simulink library "inp"  (R2021b)
settings: Solver=VariableStepAuto  StartTime=0.0  StopTime=10.0  RelTol=1e-3
undefined symbols (not defined in the file): C_TASK_5MS_S, FALSE, KINP_AcoreReadyToSlp_flg_ovrdflg, KINP_AcoreReadyToSlp_flg_ovrdval, KINP_AllowMovThd_OTA_enum_ovrdflg, KINP_AllowMovThd_OTA_enum_ovrdval, KINP_APSAngleTarget_Deg_ovrdflg, KINP_APSAngleTarget_Deg_ovrdval, KINP_APSDecReq_mps2_ovrdflg, KINP_APSDecReq_mps2_ovrdval, KINP_APSDecReqA_flg_ovrdflg, KINP_APSDecReqA_flg_ovrdval, KINP_APSDFLL_cm_ovrdflg, KINP_APSDFLL_cm_ovrdval, KINP_APSDFLR_cm_ovrdflg, KINP_APSDFLR_cm_ovrdval, KINP_APSDRLL_cm_ovrdflg, KINP_APSDRLL_cm_ovrdval, KINP_APSDRLR_cm_ovrdflg, KINP_APSDRLR_cm_ovrdval, KINP_APSExitCondition_enum_ovrdflg, KINP_APSExitCondition_enum_ovrdval, KINP_APSHWVer_enum_ovrdflg, KINP_APSHWVer_enum_ovrdval, KINP_APSProgressPCT_pct_ovrdflg, KINP_APSProgressPCT_pct_ovrdval, KINP_APSReq_enum_ovrdflg, KINP_APSReq_enum_ovrdval, KINP_APSRQDisplay_enum_ovrdflg, KINP_APSRQDisplay_enum_ovrdval, KINP_APSRqEPASCtrl_flg_ovrdflg, KINP_APSRqEPASCtrl_flg_ovrdval, KINP_APSShiftPosnReq_enum_ovrdval, KINP_APSShiftPosnReq_enum_ovrflg, KINP_APSSpeedCMD_kph_ovrdval, KINP_APSSpeedCMD_kph_ovrflg, KINP_APSStaSystem_enum_ovrdflg, KINP_APSStaSystem_enum_ovrdval, KINP_APSSWVer_enum_ovrdflg, KINP_APSSWVer_enum_ovrdval, KINP_APSVMCReqA_flg_ovrdval, KINP_APSVMCReqA_flg_ovrflg, KINP_APSVRqEPASCtrl_flg_ovrdflg, KINP_APSVRqEPASCtrl_flg_ovrdval, KINP_AuxBattVolmV_mV_ovrdflg, KINP_AuxBattVolmV_mV_ovrdval, KINP_CAASSta_enum_ovrdflg, KINP_CAASSta_enum_ovrdval, KINP_CAASVMCReqA_flg_ovrdval, KINP_CAASVMCReqA_flg_ovrflg, KINP_Chime_enum_ovrdflg, KINP_Chime_enum_ovrdval, KINP_ClearDTCcmd_flg_ovrdflg, KINP_ClearDTCcmd_flg_ovrdval, KINP_EvccAplusPwrUpReq_flg_ovrdflg, KINP_EvccAplusPwrUpReq_flg_ovrdval, KINP_LFID_raw_ovrdval, KINP_LFID_raw_ovrflg, KINP_LRID_raw_ovrdval, KINP_MemOffsetAccX_raw16_ovrdflg ... (+118)
libraries: FVT_lib x503, hcu_lib x1
(part 5 of 16)

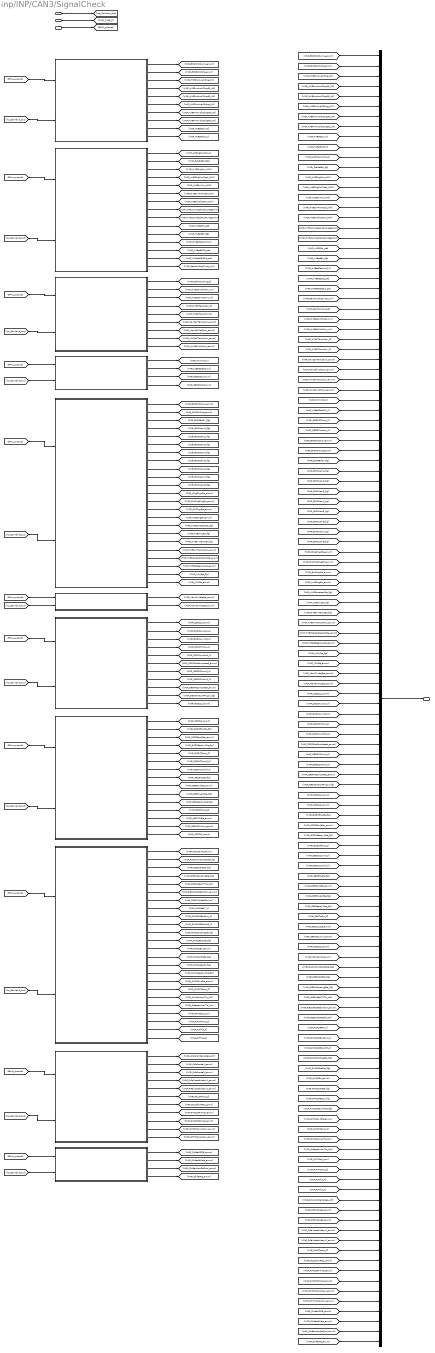
== system inp/INP/CAN3/SignalCheck ==
  inp_CanValid_bus : Inport
  TASK_TIME_S : Inport  Port=2
  BHAL_outputs : Inport  Port=3
  BMS1 : Subsystem
  BMS3 : Subsystem
  BMS4 : Subsystem
  BMS5 : Subsystem
  BMS6 : Subsystem
  BMS8 : Subsystem
  CCU1 : Subsystem
  CCU2 : Subsystem
  MCU_B_R1 : Subsystem
  MCU_B_R2 : Subsystem
  Shifter1 : Subsystem
  bus_creator : BusCreator  Inputs=128
  inp_Hal_bus : Outport
  wires:
  inp_CanValid_bus/1 -> [inp_CanValid_bus]
  TASK_TIME_S/1 -> [TASK_TIME_S]
  BHAL_outputs/1 -> [BHAL_outputs]
  [BHAL_outputs] -> BMS1/1(BHAL_outputs)
  [inp_CanValid_bus] -> BMS1/2(inp_CanValid_bus)
  BMS1/1(VINP_BMSChckSum1_enum) -> [VINP_BMSChckSum1_enum]
  BMS1/2(VINP_BMSRolCnct1_enum) -> [VINP_BMSRolCnct1_enum]
  BMS1/3(VINP_HVBPwrAvailChrg_kW) -> [VINP_HVBPwrAvailChrg_kW]
  BMS1/4(VINP_HVBPwrAvailChrg30_kW) -> [VINP_HVBPwrAvailChrg30_kW]
  BMS1/5(VINP_HVBPwrAvailChrg60_kW) -> [VINP_HVBPwrAvailChrg60_kW]
  BMS1/6(VINP_HVBPwrAvailDchrg_kW) -> [VINP_HVBPwrAvailDchrg_kW]
  BMS1/7(VINP_HVBPwrAvailDchrg30_kW) -> [VINP_HVBPwrAvailDchrg30_kW]
  BMS1/8(VINP_HVBPwrAvailDchrg60_kW) -> [VINP_HVBPwrAvailDchrg60_kW]
  BMS1/9(VINP_HVBattCurr_A) -> [VINP_HVBattCurr_A]
  BMS1/10(VINP_HVBattVolt_V) -> [VINP_HVBattVolt_V]
  [BHAL_outputs] -> BMS3/1(BHAL_outputs)
  [inp_CanValid_bus] -> BMS3/2(inp_CanValid_bus)
  BMS3/1(VINP_ACChrgCurrDis_A) -> [VINP_ACChrgCurrDis_A]
  BMS3/2(VINP_FireDetErr_flg) -> [VINP_FireDetErr_flg]
  BMS3/3(VINP_HVBChrgPwr_kWh) -> [VINP_HVBChrgPwr_kWh]
  BMS3/4(VINP_HVBChrgPwrTotal_kWh) -> [VINP_HVBChrgPwrTotal_kWh]
  BMS3/5(VINP_HVBDrvPwr_kWh) -> [VINP_HVBDrvPwr_kWh]
  BMS3/6(VINP_HVBDrvPwrTotal_kWh) -> [VINP_HVBDrvPwrTotal_kWh]
  BMS3/7(VINP_HVBFullChrgPwr_kWh) -> [VINP_HVBFullChrgPwr_kWh]
  BMS3/8(VINP_HVBIsoImpedenceN_Megaohm) -> [VINP_HVBIsoImpedenceN_Megaohm]
  BMS3/9(VINP_HVBIsoImpedenceP_Megaohm) -> [VINP_HVBIsoImpedenceP_Megaohm]
  BMS3/10(VINP_HVBSOH_pct) -> [VINP_HVBSOH_pct]
  BMS3/11(VINP_HVBattErr_flg) -> [VINP_HVBattErr_flg]
  BMS3/12(VINP_HVBattPackVolt_V) -> [VINP_HVBattPackVolt_V]
  BMS3/13(VINP_HVBattSOC_pct) -> [VINP_HVBattSOC_pct]
  BMS3/14(VINP_HVBattSOCDis_pct) -> [VINP_HVBattSOCDis_pct]
  BMS3/15(VINP_RemainChrgTime_min) -> [VINP_RemainChrgTime_min]
  [BHAL_outputs] -> BMS4/1(BHAL_outputs)
  [inp_CanValid_bus] -> BMS4/2(inp_CanValid_bus)
  BMS4/1(VINP_CellTempAvg_C) -> [VINP_CellTempAvg_C]
  BMS4/2(VINP_HVBCellVoltMax_mV) -> [VINP_HVBCellVoltMax_mV]
  BMS4/3(VINP_HVBCellVoltMin_mV) -> [VINP_HVBCellVoltMin_mV]
  BMS4/4(VINP_HVBMTempMax_C) -> [VINP_HVBMTempMax_C]
  BMS4/5(VINP_HVBMTempMin_C) -> [VINP_HVBMTempMin_C]
  BMS4/6(VINP_MaxCellTempNum_enum) -> [VINP_MaxCellTempNum_enum]
  BMS4/7(VINP_MaxCellVoltNum_enum) -> [VINP_MaxCellVoltNum_enum]
  BMS4/8(VINP_MinCellTempNum_enum) -> [VINP_MinCellTempNum_enum]
  BMS4/9(VINP_MinCellVoltNum_enum) -> [VINP_MinCellVoltNum_enum]
  [BHAL_outputs] -> BMS5/1(BHAL_outputs)
  [inp_CanValid_bus] -> BMS5/2(inp_CanValid_bus)
  BMS5/1(VINP_HVInVolt_V) -> [VINP_HVInVolt_V]
  BMS5/2(VINP_LVBattDet12V_V) -> [VINP_LVBattDet12V_V]
  BMS5/3(VINP_OBCDCCurLm_A) -> [VINP_OBCDCCurLm_A]
  BMS5/4(VINP_OBCDCVoltLm_V) -> [VINP_OBCDCVoltLm_V]
  [BHAL_outputs] -> BMS6/1(BHAL_outputs)
  [inp_CanValid_bus] -> BMS6/2(inp_CanValid_bus)
  BMS6/1(VINP_BMSChckSum_enum) -> [VINP_BMSChckSum_enum]
  BMS6/2(VINP_BMSRolCnct_enum) -> [VINP_BMSRolCnct_enum]
  BMS6/3(VINP_BMSREADY_flg) -> [VINP_BMSREADY_flg]
  BMS6/4(VINP_BMSWarn1_flg) -> [VINP_BMSWarn1_flg]
  BMS6/5(VINP_BMSWarn2_flg) -> [VINP_BMSWarn2_flg]
  BMS6/6(VINP_BMSWarn3_flg) -> [VINP_BMSWarn3_flg]
  BMS6/7(VINP_BMSWarn4_flg) -> [VINP_BMSWarn4_flg]
  BMS6/8(VINP_BMSWarn5_flg) -> [VINP_BMSWarn5_flg]
  BMS6/9(VINP_BMSWarn6_flg) -> [VINP_BMSWarn6_flg]
  BMS6/10(VINP_BMSWarn7_flg) -> [VINP_BMSWarn7_flg]
  BMS6/11(VINP_BMSWarn8_flg) -> [VINP_BMSWarn8_flg]
  BMS6/12(VINP_ChrgPlugSta_enum) -> [VINP_ChrgPlugSta_enum]
  BMS6/13(VINP_DisChrgPlugErr_enum) -> [VINP_DisChrgPlugErr_enum]
  BMS6/14(VINP_ExtChrgSta_enum) -> [VINP_ExtChrgSta_enum]
  BMS6/15(VINP_HVBChrgErr_enum) -> [VINP_HVBChrgErr_enum]
  BMS6/16(VINP_HVBContactorSta_flg) -> [VINP_HVBContactorSta_flg]
  BMS6/17(VINP_HVBHVILErr_flg) -> [VINP_HVBHVILErr_flg]
  BMS6/18(VINP_HVBOvrTempErr_flg) -> [VINP_HVBOvrTempErr_flg]
  BMS6/19(VINP_HVBOvrTempWarn_enum) -> [VINP_HVBOvrTempWarn_enum]
  BMS6/20(VINP_HVBPreheatPrecoolSta_enum) -> [VINP_HVBPreheatPrecoolSta_enum]
  BMS6/21(VINP_HVBattReady4Pre_enum) -> [VINP_HVBattReady4Pre_enum]
  BMS6/22(VINP_HVILSta_flg) -> [VINP_HVILSta_flg]
  BMS6/23(VINP_V2LSta_enum) -> [VINP_V2LSta_enum]
  [BHAL_outputs] -> BMS8/1(BHAL_outputs)
  [inp_CanValid_bus] -> BMS8/2(inp_CanValid_bus)
  BMS8/1(VINP_MainRlyNegSta_enum) -> [VINP_MainRlyNegSta_enum]
  BMS8/2(VINP_MainRlyPosSta_enum) -> [VINP_MainRlyPosSta_enum]
  [BHAL_outputs] -> CCU1/1(BHAL_outputs)
  [inp_CanValid_bus] -> CCU1/2(inp_CanValid_bus)
  CCU1/1(VINP_CSCCU1_enum) -> [VINP_CSCCU1_enum]
  CCU1/2(VINP_DCDCAuxCur_A) -> [VINP_DCDCAuxCur_A]
  CCU1/3(VINP_DCDCAuxVolt_V) -> [VINP_DCDCAuxVolt_V]
  CCU1/4(VINP_DCDCHVCur_A) -> [VINP_DCDCHVCur_A]
  CCU1/5(VINP_DCDCInVoltInf_V) -> [VINP_DCDCInVoltInf_V]
  CCU1/6(VINP_DCDCPreCompleted_enum) -> [VINP_DCDCPreCompleted_enum]
  CCU1/7(VINP_OBCDCCurrInf_A) -> [VINP_OBCDCCurrInf_A]
  CCU1/8(VINP_OBCDCVoltInf_V) -> [VINP_OBCDCVoltInf_V]
  CCU1/9(VINP_OBCPreCompleted_enum) -> [VINP_OBCPreCompleted_enum]
  CCU1/10(VINP_OBCWakeup4Plugin_flg) -> [VINP_OBCWakeup4Plugin_flg]
  CCU1/11(VINP_RCCCU1_enum) -> [VINP_RCCCU1_enum]
  [BHAL_outputs] -> CCU2/1(BHAL_outputs)
  [inp_CanValid_bus] -> CCU2/2(inp_CanValid_bus)
  CCU2/1(VINP_CSCCU2_enum) -> [VINP_CSCCU2_enum]
  CCU2/2(VINP_DCDCEnaSta_flg) -> [VINP_DCDCEnaSta_flg]
  CCU2/3(VINP_DCDCFaultSta_enum) -> [VINP_DCDCFaultSta_enum]
  CCU2/4(VINP_DCDCReady4Pre_flg) -> [VINP_DCDCReady4Pre_flg]
  CCU2/5(VINP_DCDCTemp_C) -> [VINP_DCDCTemp_C]
  CCU2/6(VINP_OBCACCurrInf_A) -> [VINP_OBCACCurrInf_A]
  CCU2/7(VINP_OBCACVoltInf_V) -> [VINP_OBCACVoltInf_V]
  CCU2/8(VINP_OBCEnaSta_flg) -> [VINP_OBCEnaSta_flg]
  CCU2/9(VINP_OBCFaultSta_enum) -> [VINP_OBCFaultSta_enum]
  CCU2/10(VINP_OBCPluginSta_flg) -> [VINP_OBCPluginSta_flg]
  CCU2/11(VINP_OBCReady4Pre_flg) -> [VINP_OBCReady4Pre_flg]
  CCU2/12(VINP_OBCTemp_C) -> [VINP_OBCTemp_C]
  CCU2/13(VINP_OBCV2LSta_enum) -> [VINP_OBCV2LSta_enum]
  CCU2/14(VINP_OBCACCurLim_enum) -> [VINP_OBCACCurLim_enum]
  CCU2/15(VINP_RCCCU2_enum) -> [VINP_RCCCU2_enum]
  [BHAL_outputs] -> MCU_B_R1/1(BHAL_outputs)
  [inp_CanValid_bus] -> MCU_B_R1/2(inp_CanValid_bus)
  MCU_B_R1/1(VINP_MCUWarnR_enum) -> [VINP_MCUWarnR_enum]
  MCU_B_R1/2(VINP_RrActvDmpDisabSta_flg) -> [VINP_RrActvDmpDisabSta_flg]
  MCU_B_R1/3(VINP_RrEDUDrtSta_flg) -> [VINP_RrEDUDrtSta_flg]
  MCU_B_R1/4(VINP_RrEDUOpratingSta_flg) -> [VINP_RrEDUOpratingSta_flg]
  MCU_B_R1/5(VINP_RrEDURealTMTq_Nm) -> [VINP_RrEDURealTMTq_Nm]
  MCU_B_R1/6(VINP_RrEDURotateDirction_enum) -> [VINP_RrEDURotateDirction_enum]
  MCU_B_R1/7(VINP_RrEDUTqReqFbk_Nm) -> [VINP_RrEDUTqReqFbk_Nm]
  MCU_B_R1/8(VINP_RrMCUBAT_V) -> [VINP_RrMCUBAT_V]
  MCU_B_R1/9(VINP_RrMCUDCBusCurr_A) -> [VINP_RrMCUDCBusCurr_A]
  MCU_B_R1/10(VINP_RrMCUDCBusVolt_V) -> [VINP_RrMCUDCBusVolt_V]
  MCU_B_R1/11(VINP_RrMCUDischrgSta_flg) -> [VINP_RrMCUDischrgSta_flg]
  MCU_B_R1/12(VINP_RrMCUEnaSta_flg) -> [VINP_RrMCUEnaSta_flg]
  MCU_B_R1/13(VINP_RrMCUErr_enum) -> [VINP_RrMCUErr_enum]
  MCU_B_R1/14(VINP_RrMCUIGNsta_flg) -> [VINP_RrMCUIGNsta_flg]
  MCU_B_R1/15(VINP_RrMCUReady_flg) -> [VINP_RrMCUReady_flg]
  MCU_B_R1/16(VINP_RrMCUReady4Pre_flg) -> [VINP_RrMCUReady4Pre_flg]
  MCU_B_R1/17(VINP_RrMCUSysSta_enum) -> [VINP_RrMCUSysSta_enum]
  MCU_B_R1/18(VINP_RrMCUTemp_C) -> [VINP_RrMCUTemp_C]
  MCU_B_R1/19(VINP_RrMotorAvailTq_Nm) -> [VINP_RrMotorAvailTq_Nm]
  MCU_B_R1/20(VINP_RrRegenAvailTq_Nm) -> [VINP_RrRegenAvailTq_Nm]
  MCU_B_R1/21(VINP_RrTMSpd_rpm) -> [VINP_RrTMSpd_rpm]
  MCU_B_R1/22(VINP_RrTMTemp_C) -> [VINP_RrTMTemp_C]
  MCU_B_R1/23(VINP_RrTMid_A) -> [VINP_RrTMid_A]
  MCU_B_R1/24(VINP_RrTMiq_A) -> [VINP_RrTMiq_A]
  [BHAL_outputs] -> MCU_B_R2/1(BHAL_outputs)
  [inp_CanValid_bus] -> MCU_B_R2/2(inp_CanValid_bus)
  MCU_B_R2/1(VINP_RrCoolanttempReq_cnt) -> [VINP_RrCoolanttempReq_cnt]
  MCU_B_R2/2(VINP_RrFailcode1_enum) -> [VINP_RrFailcode1_enum]
  MCU_B_R2/3(VINP_RrFailcode2_enum) -> [VINP_RrFailcode2_enum]
  MCU_B_R2/4(VINP_RrFailcodehistory1_enum) -> [VINP_RrFailcodehistory1_enum]
  MCU_B_R2/5(VINP_RrFailcodehistory2_enum) -> [VINP_RrFailcodehistory2_enum]
  MCU_B_R2/6(VINP_RrLLCTemp_C) -> [VINP_RrLLCTemp_C]
  MCU_B_R2/7(VINP_RrLLCflowReq_Lpmin) -> [VINP_RrLLCflowReq_Lpmin]
  MCU_B_R2/8(VINP_RrMCU3HWVer_enum) -> [VINP_RrMCU3HWVer_enum]
  MCU_B_R2/9(VINP_RrMCU3SWVer_enum) -> [VINP_RrMCU3SWVer_enum]
  MCU_B_R2/10(VINP_RrMCUTempWarn_enum) -> [VINP_RrMCUTempWarn_enum]
  MCU_B_R2/11(VINP_RrTMTempWarn_enum) -> [VINP_RrTMTempWarn_enum]
  [BHAL_outputs] -> Shifter1/1(BHAL_outputs)
  [inp_CanValid_bus] -> Shifter1/2(inp_CanValid_bus)
  Shifter1/1(VINP_ShifterCRC8_enum) -> [VINP_ShifterCRC8_enum]
  Shifter1/2(VINP_ShifterFailsta_enum) -> [VINP_ShifterFailsta_enum]
  Shifter1/3(VINP_ShifterHandleCmd_enum) -> [VINP_ShifterHandleCmd_enum]
  Shifter1/4(VINP_ShifterRC_enum) -> [VINP_ShifterRC_enum]
  bus_creator/1 -> inp_Hal_bus/1
  [VINP_BMSChckSum1_enum] -> bus_creator/1
  [VINP_BMSRolCnct1_enum] -> bus_creator/2
  [VINP_HVBPwrAvailChrg_kW] -> bus_creator/3
  [VINP_HVBPwrAvailChrg30_kW] -> bus_creator/4
  [VINP_HVBPwrAvailChrg60_kW] -> bus_creator/5
  [VINP_HVBPwrAvailDchrg_kW] -> bus_creator/6
  [VINP_HVBPwrAvailDchrg30_kW] -> bus_creator/7
  [VINP_HVBPwrAvailDchrg60_kW] -> bus_creator/8
  [VINP_HVBattCurr_A] -> bus_creator/9
  [VINP_HVBattVolt_V] -> bus_creator/10
  [VINP_ACChrgCurrDis_A] -> bus_creator/11
  [VINP_FireDetErr_flg] -> bus_creator/12
  [VINP_HVBChrgPwr_kWh] -> bus_creator/13
  [VINP_HVBChrgPwrTotal_kWh] -> bus_creator/14
  [VINP_HVBDrvPwr_kWh] -> bus_creator/15
  [VINP_HVBDrvPwrTotal_kWh] -> bus_creator/16
  [VINP_HVBFullChrgPwr_kWh] -> bus_creator/17
  [VINP_HVBIsoImpedenceN_Megaohm] -> bus_creator/18
  [VINP_HVBIsoImpedenceP_Megaohm] -> bus_creator/19
  [VINP_HVBSOH_pct] -> bus_creator/20
  [VINP_HVBattErr_flg] -> bus_creator/21
  [VINP_HVBattPackVolt_V] -> bus_creator/22
  [VINP_HVBattSOC_pct] -> bus_creator/23
  [VINP_HVBattSOCDis_pct] -> bus_creator/24
  [VINP_RemainChrgTime_min] -> bus_creator/25
  [VINP_CellTempAvg_C] -> bus_creator/26
  [VINP_HVBCellVoltMax_mV] -> bus_creator/27
  [VINP_HVBCellVoltMin_mV] -> bus_creator/28
  [VINP_HVBMTempMax_C] -> bus_creator/29
  [VINP_HVBMTempMin_C] -> bus_creator/30
  [VINP_MaxCellTempNum_enum] -> bus_creator/31
  [VINP_MaxCellVoltNum_enum] -> bus_creator/32
  [VINP_MinCellTempNum_enum] -> bus_creator/33
  [VINP_MinCellVoltNum_enum] -> bus_creator/34
  [VINP_HVInVolt_V] -> bus_creator/35
  [VINP_LVBattDet12V_V] -> bus_creator/36
  [VINP_OBCDCCurLm_A] -> bus_creator/37
  [VINP_OBCDCVoltLm_V] -> bus_creator/38
  [VINP_BMSChckSum_enum] -> bus_creator/39
  [VINP_BMSRolCnct_enum] -> bus_creator/40
  [VINP_BMSREADY_flg] -> bus_creator/41
  [VINP_BMSWarn1_flg] -> bus_creator/42
  [VINP_BMSWarn2_flg] -> bus_creator/43
  [VINP_BMSWarn3_flg] -> bus_creator/44
  [VINP_BMSWarn4_flg] -> bus_creator/45
  [VINP_BMSWarn5_flg] -> bus_creator/46
  [VINP_BMSWarn6_flg] -> bus_creator/47
  [VINP_BMSWarn7_flg] -> bus_creator/48
  [VINP_BMSWarn8_flg] -> bus_creator/49
  [VINP_ChrgPlugSta_enum] -> bus_creator/50
  [VINP_DisChrgPlugErr_enum] -> bus_creator/51
  [VINP_ExtChrgSta_enum] -> bus_creator/52
  [VINP_HVBChrgErr_enum] -> bus_creator/53
  [VINP_HVBContactorSta_flg] -> bus_creator/54
  [VINP_HVBHVILErr_flg] -> bus_creator/55
  [VINP_HVBOvrTempErr_flg] -> bus_creator/56
  [VINP_HVBOvrTempWarn_enum] -> bus_creator/57
  [VINP_HVBPreheatPrecoolSta_enum] -> bus_creator/58
  [VINP_HVBattReady4Pre_enum] -> bus_creator/59
  [VINP_HVILSta_flg] -> bus_creator/60
  [VINP_V2LSta_enum] -> bus_creator/61
  [VINP_MainRlyNegSta_enum] -> bus_creator/62
  [VINP_MainRlyPosSta_enum] -> bus_creator/63
  [VINP_CSCCU1_enum] -> bus_creator/64
  [VINP_DCDCAuxCur_A] -> bus_creator/65
  [VINP_DCDCAuxVolt_V] -> bus_creator/66
  [VINP_DCDCHVCur_A] -> bus_creator/67
  [VINP_DCDCInVoltInf_V] -> bus_creator/68
  [VINP_DCDCPreCompleted_enum] -> bus_creator/69
  [VINP_OBCDCCurrInf_A] -> bus_creator/70
  [VINP_OBCDCVoltInf_V] -> bus_creator/71
  [VINP_OBCPreCompleted_enum] -> bus_creator/72
  [VINP_OBCWakeup4Plugin_flg] -> bus_creator/73
  [VINP_RCCCU1_enum] -> bus_creator/74
  [VINP_CSCCU2_enum] -> bus_creator/75
  [VINP_DCDCEnaSta_flg] -> bus_creator/76
  [VINP_DCDCFaultSta_enum] -> bus_creator/77
  [VINP_DCDCReady4Pre_flg] -> bus_creator/78
  [VINP_DCDCTemp_C] -> bus_creator/79
  [VINP_OBCACCurrInf_A] -> bus_creator/80
  [VINP_OBCACVoltInf_V] -> bus_creator/81
  [VINP_OBCEnaSta_flg] -> bus_creator/82
  [VINP_OBCFaultSta_enum] -> bus_creator/83
  [VINP_OBCPluginSta_flg] -> bus_creator/84
  [VINP_OBCReady4Pre_flg] -> bus_creator/85
  [VINP_OBCTemp_C] -> bus_creator/86
  [VINP_OBCV2LSta_enum] -> bus_creator/87
  [VINP_OBCACCurLim_enum] -> bus_creator/88
  [VINP_RCCCU2_enum] -> bus_creator/89
  [VINP_MCUWarnR_enum] -> bus_creator/90
  [VINP_RrActvDmpDisabSta_flg] -> bus_creator/91
  [VINP_RrEDUDrtSta_flg] -> bus_creator/92
  [VINP_RrEDUOpratingSta_flg] -> bus_creator/93
  [VINP_RrEDURealTMTq_Nm] -> bus_creator/94
  [VINP_RrEDURotateDirction_enum] -> bus_creator/95
  [VINP_RrEDUTqReqFbk_Nm] -> bus_creator/96
  [VINP_RrMCUBAT_V] -> bus_creator/97
  [VINP_RrMCUDCBusCurr_A] -> bus_creator/98
  [VINP_RrMCUDCBusVolt_V] -> bus_creator/99
  [VINP_RrMCUDischrgSta_flg] -> bus_creator/100
  [VINP_RrMCUEnaSta_flg] -> bus_creator/101
  [VINP_RrMCUErr_enum] -> bus_creator/102
  [VINP_RrMCUIGNsta_flg] -> bus_creator/103
  [VINP_RrMCUReady_flg] -> bus_creator/104
  [VINP_RrMCUReady4Pre_flg] -> bus_creator/105
  [VINP_RrMCUSysSta_enum] -> bus_creator/106
  [VINP_RrMCUTemp_C] -> bus_creator/107
  [VINP_RrMotorAvailTq_Nm] -> bus_creator/108
  [VINP_RrRegenAvailTq_Nm] -> bus_creator/109
  [VINP_RrTMSpd_rpm] -> bus_creator/110
  [VINP_RrTMTemp_C] -> bus_creator/111
  [VINP_RrTMid_A] -> bus_creator/112
  [VINP_RrTMiq_A] -> bus_creator/113
  [VINP_RrCoolanttempReq_cnt] -> bus_creator/114
  [VINP_RrFailcode1_enum] -> bus_creator/115
  [VINP_RrFailcode2_enum] -> bus_creator/116
  [VINP_RrFailcodehistory1_enum] -> bus_creator/117
  [VINP_RrFailcodehistory2_enum] -> bus_creator/118
  [VINP_RrLLCTemp_C] -> bus_creator/119
  [VINP_RrLLCflowReq_Lpmin] -> bus_creator/120
  [VINP_RrMCU3HWVer_enum] -> bus_creator/121
  [VINP_RrMCU3SWVer_enum] -> bus_creator/122
  [VINP_RrMCUTempWarn_enum] -> bus_creator/123
  [VINP_RrTMTempWarn_enum] -> bus_creator/124
  [VINP_ShifterCRC8_enum] -> bus_creator/125
  [VINP_ShifterFailsta_enum] -> bus_creator/126
  [VINP_ShifterHandleCmd_enum] -> bus_creator/127
  [VINP_ShifterRC_enum] -> bus_creator/128

== system inp/INP/CAN4/CommunicationCheck ==
  BHAL_outputs : Inport
  CANMsgInvalidDKC1 : FVT_lib/inp/CAN_Msg_Validity_Process_template  SystemSampleTime=-1  VariantActivationTime=update diagram  Latency=0  AutoFrameSizeCalculation=off
      link override ovrdflg: Value=KINP_CANMsgInvalidDKC1_flg_ovrdflg
      link override ovrdval: Value=KINP_CANMsgInvalidDKC1_flg_ovrdval
  CANMsgInvalidDKC2 : FVT_lib/inp/CAN_Msg_Validity_Process_template  SystemSampleTime=-1  VariantActivationTime=update diagram  Latency=0  AutoFrameSizeCalculation=off
      link override ovrdflg: Value=KINP_CANMsgInvalidDKC2_flg_ovrdflg
      link override ovrdval: Value=KINP_CANMsgInvalidDKC2_flg_ovrdval
  CANMsgInvalidZ24C10000 : FVT_lib/inp/CAN_Msg_Validity_Process_template  SystemSampleTime=-1  VariantActivationTime=update diagram  Latency=0  AutoFrameSizeCalculation=off
      link override ovrdflg: Value=KINP_CANMsgInvalidZ24C10000_flg_ovrdflg
      link override ovrdval: Value=KINP_CANMsgInvalidZ24C10000_flg_ovrdval
  CANMsgInvalidZ24CE1000 : FVT_lib/inp/CAN_Msg_Validity_Process_template  SystemSampleTime=-1  VariantActivationTime=update diagram  Latency=0  AutoFrameSizeCalculation=off
      link override ovrdflg: Value=KINP_CANMsgInvalidZ24CE1000_flg_ovrdflg
      link override ovrdval: Value=KINP_CANMsgInvalidZ24CE1000_flg_ovrdval
  CANMsgInvalidZONEDR1 : FVT_lib/inp/CAN_Msg_Validity_Process_template  SystemSampleTime=-1  VariantActivationTime=update diagram  Latency=0  AutoFrameSizeCalculation=off
      link override ovrdflg: Value=KINP_CANMsgInvalidZONEDR1_flg_ovrdflg
      link override ovrdval: Value=KINP_CANMsgInvalidZONEDR1_flg_ovrdval
  CANMsgInvalidZONEDRVCU : FVT_lib/inp/CAN_Msg_Validity_Process_template  SystemSampleTime=-1  VariantActivationTime=update diagram  Latency=0  AutoFrameSizeCalculation=off
      link override ovrdflg: Value=KINP_CANMsgInvalidZONEDRVCU_flg_ovrdflg
      link override ovrdval: Value=KINP_CANMsgInvalidZONEDRVCU_flg_ovrdval
  CANMsgInvalidZONEFR1 : FVT_lib/inp/CAN_Msg_Validity_Process_template  SystemSampleTime=-1  VariantActivationTime=update diagram  Latency=0  AutoFrameSizeCalculation=off
      link override ovrdflg: Value=KINP_CANMsgInvalidZONEFR1_flg_ovrdflg
      link override ovrdval: Value=KINP_CANMsgInvalidZONEFR1_flg_ovrdval
  CANMsgInvalidZONEFRVCU : FVT_lib/inp/CAN_Msg_Validity_Process_template  SystemSampleTime=-1  VariantActivationTime=update diagram  Latency=0  AutoFrameSizeCalculation=off
      link override ovrdflg: Value=KINP_CANMsgInvalidZONEFRVCU_flg_ovrdflg
      link override ovrdval: Value=KINP_CANMsgInvalidZONEFRVCU_flg_ovrdval
  CANMsgInvalidzGWAPTC1 : FVT_lib/inp/CAN_Msg_Validity_Process_template  SystemSampleTime=-1  VariantActivationTime=update diagram  Latency=0  AutoFrameSizeCalculation=off
      link override ovrdflg: Value=KINP_CANMsgInvalidzGWAPTC1_flg_ovrdflg
      link override ovrdval: Value=KINP_CANMsgInvalidzGWAPTC1_flg_ovrdval
  CANMsgInvalidzGWCANFr1 : FVT_lib/inp/CAN_Msg_Validity_Process_template  SystemSampleTime=-1  VariantActivationTime=update diagram  Latency=0  AutoFrameSizeCalculation=off
      link override ovrdflg: Value=KINP_CANMsgInvalidzGWCANFr1_flg_ovrdflg
      link override ovrdval: Value=KINP_CANMsgInvalidzGWCANFr1_flg_ovrdval
  CANMsgInvalidzGWLINDr1 : FVT_lib/inp/CAN_Msg_Validity_Process_template  SystemSampleTime=-1  VariantActivationTime=update diagram  Latency=0  AutoFrameSizeCalculation=off
      link override ovrdflg: Value=KINP_CANMsgInvalidzGWLINDr1_flg_ovrdflg
      link override ovrdval: Value=KINP_CANMsgInvalidzGWLINDr1_flg_ovrdval
  bus_creator : BusCreator  Inputs=11
  bus_selector : BusSelector  OutputSignals=VHAL_CANMsgInvalidDKC1_flg,VHAL_CANMsgInvalidDKC2_flg,VHAL_CANMsgInvalidZ24C10000_flg,VHAL_CANMsgInvalidZ24CE1000_flg,VHAL_CANMsgInvalidZONEDR1_flg,VHAL_CANMsgInvalidZONEDRVCU_flg,VHAL_CANMsgInvalidZONEFR1_flg,VHAL_CANMsgInvalidZONEFRVCU_flg,VHAL_CANMsgInvalidzGWAPTC1_flg,VHAL_CANMsgInvalidzGWCANFr1_flg,VHAL_CANMsgInvalidzGWLINDr1_flg
  not{1..11} (11 alike) : Logic  Operator=NOT  AllPortsSameDT=off  OutDataTypeStr=boolean
  inp_CanValid_bus : Outport
  wires:
  BHAL_outputs/1 -> [BHAL_outputs]
  bus_selector/1 -> CANMsgInvalidDKC1/1  "<VHAL_CANMsgInvalidDKC1_flg>"
  CANMsgInvalidDKC1/1 -> not1/1
  not1/1 -> bus_creator/1  "VINP_CANMsgValidDKC1_flg"
  bus_selector/2 -> CANMsgInvalidDKC2/1  "<VHAL_CANMsgInvalidDKC2_flg>"
  CANMsgInvalidDKC2/1 -> not2/1
  not2/1 -> bus_creator/2  "VINP_CANMsgValidDKC2_flg"
  bus_selector/3 -> CANMsgInvalidZ24C10000/1  "<VHAL_CANMsgInvalidZ24C10000_flg>"
  CANMsgInvalidZ24C10000/1 -> not3/1
  not3/1 -> bus_creator/3  "VINP_CANMsgValidZ24C10000_flg"
  bus_selector/4 -> CANMsgInvalidZ24CE1000/1  "<VHAL_CANMsgInvalidZ24CE1000_flg>"
  CANMsgInvalidZ24CE1000/1 -> not4/1
  not4/1 -> bus_creator/4  "VINP_CANMsgValidZ24CE1000_flg"
  bus_selector/5 -> CANMsgInvalidZONEDR1/1  "<VHAL_CANMsgInvalidZONEDR1_flg>"
  CANMsgInvalidZONEDR1/1 -> not5/1
  not5/1 -> bus_creator/5  "VINP_CANMsgValidZONEDR1_flg"
  bus_selector/6 -> CANMsgInvalidZONEDRVCU/1  "<VHAL_CANMsgInvalidZONEDRVCU_flg>"
  CANMsgInvalidZONEDRVCU/1 -> not6/1
  not6/1 -> bus_creator/6  "VINP_CANMsgValidZONEDRVCU_flg"
  bus_selector/7 -> CANMsgInvalidZONEFR1/1  "<VHAL_CANMsgInvalidZONEFR1_flg>"
  CANMsgInvalidZONEFR1/1 -> not7/1
  not7/1 -> bus_creator/7  "VINP_CANMsgValidZONEFR1_flg"
  bus_selector/8 -> CANMsgInvalidZONEFRVCU/1  "<VHAL_CANMsgInvalidZONEFRVCU_flg>"
  CANMsgInvalidZONEFRVCU/1 -> not8/1
  not8/1 -> bus_creator/8  "VINP_CANMsgValidZONEFRVCU_flg"
  bus_selector/9 -> CANMsgInvalidzGWAPTC1/1  "<VHAL_CANMsgInvalidzGWAPTC1_flg>"
  CANMsgInvalidzGWAPTC1/1 -> not9/1
  not9/1 -> bus_creator/9  "VINP_CANMsgValidzGWAPTC1_flg"
  bus_selector/10 -> CANMsgInvalidzGWCANFr1/1  "<VHAL_CANMsgInvalidzGWCANFr1_flg>"
  CANMsgInvalidzGWCANFr1/1 -> not10/1
  not10/1 -> bus_creator/10  "VINP_CANMsgValidzGWCANFr1_flg"
  bus_selector/11 -> CANMsgInvalidzGWLINDr1/1  "<VHAL_CANMsgInvalidzGWLINDr1_flg>"
  CANMsgInvalidzGWLINDr1/1 -> not11/1
  not11/1 -> bus_creator/11  "VINP_CANMsgValidzGWLINDr1_flg"
  [BHAL_outputs] -> bus_selector/1
  bus_creator/1 -> inp_CanValid_bus/1

== system inp/INP/CAN4/CreateBus ==
  inp_CanValid_bus : Inport
  inp_Hal_bus : Inport  Port=2
  UnitConverter_{1..11,20,22,29..32,35..36,38..41,63..64,67..69,80,110,113,117..119,121..122,124..125,127..128,130..131,133..147} (57 alike) : DataTypeConversion  OutDataTypeStr=boolean
  UnitConverter_{12..19,21,37,43,45,47,49,51,53,55,57,59,61..62,70,72,74..79,82,84,86,88,90,92,94,96..100,102,111..112,114..116,132} (48 alike) : DataTypeConversion  OutDataTypeStr=uint8
  UnitConverter_{26..28,33..34,42,44,46,48,50,52,54,56,58,60,65..66,71,73,81,83,85,87,89,91,93,95,101,103..108,120,123,126,129} (38 alike) : DataTypeConversion  OutDataTypeStr=single
  UnitConverter_109 : DataTypeConversion  OutDataTypeStr=uint16
  UnitConverter_23 : DataTypeConversion  OutDataTypeStr=uint64
  UnitConverter_24 : DataTypeConversion  OutDataTypeStr=uint64
  UnitConverter_25 : DataTypeConversion  OutDataTypeStr=uint64
  bus_creator : BusCreator  Inputs=147
  bus_selector : BusSelector  OutputSignals=VINP_CANMsgValidDKC1_flg,VINP_CANMsgValidDKC2_flg,VINP_CANMsgValidZ24C10000_flg,VINP_CANMsgValidZ24CE1000_flg,VINP_CANMsgValidZONEDR1_flg,VINP_CANMsgValidZONEDRVCU_flg,VINP_CANMsgValidZONEFR1_flg,VINP_CANMsgValidZONEFRVCU_flg,VINP_CANMsgValidzGWAPTC1_flg,VINP_CANMsgValidzGWCANFr1_flg,VINP_CANMsgValidzGWLINDr1_flg
  bus_selector_1 : BusSelector  OutputSignals=VINP_DKCReVehData_enum,VINP_PCommandToBCM_enum,VINP_PCommandToPTG_enum,VINP_PDKeyAreaLockUnlock_enum,VINP_PDKeyAreaPS_enum,VINP_PDKeyAreaPTG_enum,VINP_PDKeyWelcome_enum,VINP_PDkeyShowIVI_enum,VINP_PKeyMiss_flg,VINP_PKeyMode_enum,VINP_PUIDLowPower_flg,VINP_EncryptionDATA063_enum,VINP_EncryptionDATA64127_enum,VINP_RandomNumberX_enum,VINP_Z24CHAAirPressureFC2Sta_KPa,VINP_Z24CHAAirPressurePC3Sta_KPa,VINP_Z24CHAAirPressureRC1Sta_KPa,VINP_Z24BCMFWiperASSta_flg,VINP_Z24BCMSeatBeltSWSta_flg,VINP_DrLockSta_flg,VINP_MIRRORFOLDSW_flg,VINP_RLTurnLampC_mA,VINP_RRTurnLampC_mA,VINP_RWiperAS_flg,VINP_RWiperProtection_flg,VINP_BlowerErr_enum,VINP_DrPMMLVOutPErrLmp_flg,VINP_DrPMMSysErrLmp_flg,VINP_DrSCPSysErrLmp_flg,VINP_DrStdAErrSta_flg,VINP_SolarL_W,VINP_SolarLErr_enum,VINP_SolarR_W,VINP_SolarRErr_enum,VINP_TFaceL_C,VINP_TFaceLErr_enum,VINP_TFaceR_C,VINP_TFaceRErr_enum,VINP_TFaceRr_C,VINP_TFaceRrErr_enum,VINP_TFootL_C,VINP_TFootLErr_enum,VINP_TFootR_C,VINP_TFootRErr_enum,VINP_TFootRr_C,VINP_TFootRrErr_enum,VINP_Tevap_C,VINP_TevapErr_enum,VINP_Tincar_C,VINP_TincarErr_enum,VINP_ZoneDrMalfunLevel_enum,VINP_ChargeInletLockSta_flg,VINP_CompProEN_flg,VINP_FLTurnLampC_mA,VINP_FRTurnLampC_mA,VINP_FWiperAS_flg,VINP_FWiperProtection_flg,VINP_TrailerCheck_flg,VINP_TrailerModeSta_enum,VINP_BatInTemp_C,VINP_BatInTempErr_enum,VINP_BatOutTemp_C,VINP_COMPErr_enum,VINP_EACProtectEnable_enum,VINP_EWP3Err_enum,VINP_EXV1Err_enum,VINP_EXV2Err_enum,VINP_FanErr_enum,VINP_FrPMMLimpHomeActReq_flg,VINP_MotorInTemp_C,VINP_MotorInTempErr_enum,VINP_MotorOutTemp_C,VINP_MotorOutTempErr_enum,VINP_PTHighP_KPa,VINP_PTHighPErr_enum,VINP_PTHighTact_C,VINP_PTHighTactErr_enum,VINP_PTLowP1_KPa,VINP_PTLowP1Err_enum,VINP_PTLowP2_KPa,VINP_PTLowP2Err_enum,VINP_PTLowT1_C,VINP_PTLowT1Err_enum,VINP_PTLowT2_C,VINP_PTLowT2Err_enum,VINP_SOTXVErr_enum,VINP_SOV1Err_enum,VINP_SOV2Err_enum,VINP_SOV3Err_enum,VINP_Tamb_C,VINP_TambErr_enum,VINP_FrntPTCLeActHeatPwr_W,VINP_FrntPTCRearLeActHeatPwr_W,VINP_FrntPTCRearRiActHeatPwr_W,VINP_FrntPTCRiActHeatPwr_W,VINP_COMPActualPwr_W,VINP_COMPStatorSpd_rpm,VINP_PTCActuPwrHSC6_enum,VINP_CSWDimSw_flg,VINP_CSWFWasSwSta_enum,VINP_CSWFWipSwSta_enum,VINP_CSWPassSWSta_flg,VINP_CSWRWasSWSta_enum,VINP_CSWRWipIntSwSta_enum,VINP_CSWTurnSwSta_enum,VINP_FAPWL01LINResponseError_flg,VINP_LDrvMotorRelayError_flg,VINP_LDrvMotorRippleError_flg,VINP_LDrvValWdwOpened_pct,VINP_LPasMotorRelayError_flg,VINP_LPasMotorRippleError_flg,VINP_LPasValWdwOpened_pct,VINP_LRLDMotorRelayError_flg,VINP_LRLDMotorRippleError_flg,VINP_LRLDValWdwOpened_pct,VINP_LRRDMotorRelayError_flg,VINP_LRRDMotorRippleError_flg,VINP_LRRDValWdwOpened_pct,VINP_RAPWL01LINResponseError_flg,VINP_RLSLampSta_flg,VINP_RLSRainSnrWiperCmd_enum,VINP_SWCACCSta_flg,VINP_SWCCANCELSta_flg,VINP_SWCDistanceSta_flg,VINP_SWCDownSta_flg,VINP_SWCLKASta_flg,VINP_SWCLeftSta_flg,VINP_SWCRegenUp_flg,VINP_SWCResUpSta_flg,VINP_SWCRightSta_flg,VINP_SWCSetdownSta_flg,VINP_SWCTripSta_flg,VINP_SWCUndefinedSta_flg,VINP_SWCUpSta_flg,VINP_SWCVRSta_flg,VINP_SWCmodeSta_flg
  BINP_outputs : Outport
  wires:
  inp_CanValid_bus/1 -> [inp_CanValid_bus]
  inp_Hal_bus/1 -> [inp_Hal_bus]
  bus_selector/1 -> UnitConverter_1/1  "<VINP_CANMsgValidDKC1_flg>"
  UnitConverter_1/1 -> bus_creator/1  "VINP_CANMsgValidDKC1_flg"
  bus_selector/2 -> UnitConverter_2/1  "<VINP_CANMsgValidDKC2_flg>"
  UnitConverter_2/1 -> bus_creator/2  "VINP_CANMsgValidDKC2_flg"
  bus_selector/3 -> UnitConverter_3/1  "<VINP_CANMsgValidZ24C10000_flg>"
  UnitConverter_3/1 -> bus_creator/3  "VINP_CANMsgValidZ24C10000_flg"
  bus_selector/4 -> UnitConverter_4/1  "<VINP_CANMsgValidZ24CE1000_flg>"
  UnitConverter_4/1 -> bus_creator/4  "VINP_CANMsgValidZ24CE1000_flg"
  bus_selector/5 -> UnitConverter_5/1  "<VINP_CANMsgValidZONEDR1_flg>"
  UnitConverter_5/1 -> bus_creator/5  "VINP_CANMsgValidZONEDR1_flg"
  bus_selector/6 -> UnitConverter_6/1  "<VINP_CANMsgValidZONEDRVCU_flg>"
  UnitConverter_6/1 -> bus_creator/6  "VINP_CANMsgValidZONEDRVCU_flg"
  bus_selector/7 -> UnitConverter_7/1  "<VINP_CANMsgValidZONEFR1_flg>"
  UnitConverter_7/1 -> bus_creator/7  "VINP_CANMsgValidZONEFR1_flg"
  bus_selector/8 -> UnitConverter_8/1  "<VINP_CANMsgValidZONEFRVCU_flg>"
  UnitConverter_8/1 -> bus_creator/8  "VINP_CANMsgValidZONEFRVCU_flg"
  bus_selector/9 -> UnitConverter_9/1  "<VINP_CANMsgValidzGWAPTC1_flg>"
  UnitConverter_9/1 -> bus_creator/9  "VINP_CANMsgValidzGWAPTC1_flg"
  bus_selector/10 -> UnitConverter_10/1  "<VINP_CANMsgValidzGWCANFr1_flg>"
  UnitConverter_10/1 -> bus_creator/10  "VINP_CANMsgValidzGWCANFr1_flg"
  bus_selector/11 -> UnitConverter_11/1  "<VINP_CANMsgValidzGWLINDr1_flg>"
  UnitConverter_11/1 -> bus_creator/11  "VINP_CANMsgValidzGWLINDr1_flg"
  bus_selector_1/1 -> UnitConverter_12/1  "<VINP_DKCReVehData_enum>"
  UnitConverter_12/1 -> bus_creator/12  "VINP_DKCReVehData_enum"
  bus_selector_1/2 -> UnitConverter_13/1  "<VINP_PCommandToBCM_enum>"
  UnitConverter_13/1 -> bus_creator/13  "VINP_PCommandToBCM_enum"
  bus_selector_1/3 -> UnitConverter_14/1  "<VINP_PCommandToPTG_enum>"
  UnitConverter_14/1 -> bus_creator/14  "VINP_PCommandToPTG_enum"
  bus_selector_1/4 -> UnitConverter_15/1  "<VINP_PDKeyAreaLockUnlock_enum>"
  UnitConverter_15/1 -> bus_creator/15  "VINP_PDKeyAreaLockUnlock_enum"
  bus_selector_1/5 -> UnitConverter_16/1  "<VINP_PDKeyAreaPS_enum>"
  UnitConverter_16/1 -> bus_creator/16  "VINP_PDKeyAreaPS_enum"
  bus_selector_1/6 -> UnitConverter_17/1  "<VINP_PDKeyAreaPTG_enum>"
  UnitConverter_17/1 -> bus_creator/17  "VINP_PDKeyAreaPTG_enum"
  bus_selector_1/7 -> UnitConverter_18/1  "<VINP_PDKeyWelcome_enum>"
  UnitConverter_18/1 -> bus_creator/18  "VINP_PDKeyWelcome_enum"
  bus_selector_1/8 -> UnitConverter_19/1  "<VINP_PDkeyShowIVI_enum>"
  UnitConverter_19/1 -> bus_creator/19  "VINP_PDkeyShowIVI_enum"
  bus_selector_1/9 -> UnitConverter_20/1  "<VINP_PKeyMiss_flg>"
  UnitConverter_20/1 -> bus_creator/20  "VINP_PKeyMiss_flg"
  bus_selector_1/10 -> UnitConverter_21/1  "<VINP_PKeyMode_enum>"
  UnitConverter_21/1 -> bus_creator/21  "VINP_PKeyMode_enum"
  bus_selector_1/11 -> UnitConverter_22/1  "<VINP_PUIDLowPower_flg>"
  UnitConverter_22/1 -> bus_creator/22  "VINP_PUIDLowPower_flg"
  bus_selector_1/12 -> UnitConverter_23/1  "<VINP_EncryptionDATA063_enum>"
  UnitConverter_23/1 -> bus_creator/23  "VINP_EncryptionDATA063_enum"
  bus_selector_1/13 -> UnitConverter_24/1  "<VINP_EncryptionDATA64127_enum>"
  UnitConverter_24/1 -> bus_creator/24  "VINP_EncryptionDATA64127_enum"
  bus_selector_1/14 -> UnitConverter_25/1  "<VINP_RandomNumberX_enum>"
  UnitConverter_25/1 -> bus_creator/25  "VINP_RandomNumberX_enum"
  bus_selector_1/15 -> UnitConverter_26/1  "<VINP_Z24CHAAirPressureFC2Sta_KPa>"
  UnitConverter_26/1 -> bus_creator/26  "VINP_Z24CHAAirPressureFC2Sta_KPa"
  bus_selector_1/16 -> UnitConverter_27/1  "<VINP_Z24CHAAirPressurePC3Sta_KPa>"
  UnitConverter_27/1 -> bus_creator/27  "VINP_Z24CHAAirPressurePC3Sta_KPa"
  bus_selector_1/17 -> UnitConverter_28/1  "<VINP_Z24CHAAirPressureRC1Sta_KPa>"
  UnitConverter_28/1 -> bus_creator/28  "VINP_Z24CHAAirPressureRC1Sta_KPa"
  bus_selector_1/18 -> UnitConverter_29/1  "<VINP_Z24BCMFWiperASSta_flg>"
  UnitConverter_29/1 -> bus_creator/29  "VINP_Z24BCMFWiperASSta_flg"
  bus_selector_1/19 -> UnitConverter_30/1  "<VINP_Z24BCMSeatBeltSWSta_flg>"
  UnitConverter_30/1 -> bus_creator/30  "VINP_Z24BCMSeatBeltSWSta_flg"
  bus_selector_1/20 -> UnitConverter_31/1  "<VINP_DrLockSta_flg>"
  UnitConverter_31/1 -> bus_creator/31  "VINP_DrLockSta_flg"
  bus_selector_1/21 -> UnitConverter_32/1  "<VINP_MIRRORFOLDSW_flg>"
  UnitConverter_32/1 -> bus_creator/32  "VINP_MIRRORFOLDSW_flg"
  bus_selector_1/22 -> UnitConverter_33/1  "<VINP_RLTurnLampC_mA>"
  UnitConverter_33/1 -> bus_creator/33  "VINP_RLTurnLampC_mA"
  bus_selector_1/23 -> UnitConverter_34/1  "<VINP_RRTurnLampC_mA>"
  UnitConverter_34/1 -> bus_creator/34  "VINP_RRTurnLampC_mA"
  bus_selector_1/24 -> UnitConverter_35/1  "<VINP_RWiperAS_flg>"
  UnitConverter_35/1 -> bus_creator/35  "VINP_RWiperAS_flg"
  bus_selector_1/25 -> UnitConverter_36/1  "<VINP_RWiperProtection_flg>"
  UnitConverter_36/1 -> bus_creator/36  "VINP_RWiperProtection_flg"
  bus_selector_1/26 -> UnitConverter_37/1  "<VINP_BlowerErr_enum>"
  UnitConverter_37/1 -> bus_creator/37  "VINP_BlowerErr_enum"
  bus_selector_1/27 -> UnitConverter_38/1  "<VINP_DrPMMLVOutPErrLmp_flg>"
  UnitConverter_38/1 -> bus_creator/38  "VINP_DrPMMLVOutPErrLmp_flg"
  bus_selector_1/28 -> UnitConverter_39/1  "<VINP_DrPMMSysErrLmp_flg>"
  UnitConverter_39/1 -> bus_creator/39  "VINP_DrPMMSysErrLmp_flg"
  bus_selector_1/29 -> UnitConverter_40/1  "<VINP_DrSCPSysErrLmp_flg>"
  UnitConverter_40/1 -> bus_creator/40  "VINP_DrSCPSysErrLmp_flg"
  bus_selector_1/30 -> UnitConverter_41/1  "<VINP_DrStdAErrSta_flg>"
  UnitConverter_41/1 -> bus_creator/41  "VINP_DrStdAErrSta_flg"
  bus_selector_1/31 -> UnitConverter_42/1  "<VINP_SolarL_W>"
  UnitConverter_42/1 -> bus_creator/42  "VINP_SolarL_W"
  bus_selector_1/32 -> UnitConverter_43/1  "<VINP_SolarLErr_enum>"
  UnitConverter_43/1 -> bus_creator/43  "VINP_SolarLErr_enum"
  bus_selector_1/33 -> UnitConverter_44/1  "<VINP_SolarR_W>"
  UnitConverter_44/1 -> bus_creator/44  "VINP_SolarR_W"
  bus_selector_1/34 -> UnitConverter_45/1  "<VINP_SolarRErr_enum>"
  UnitConverter_45/1 -> bus_creator/45  "VINP_SolarRErr_enum"
  bus_selector_1/35 -> UnitConverter_46/1  "<VINP_TFaceL_C>"
  UnitConverter_46/1 -> bus_creator/46  "VINP_TFaceL_C"
  bus_selector_1/36 -> UnitConverter_47/1  "<VINP_TFaceLErr_enum>"
  UnitConverter_47/1 -> bus_creator/47  "VINP_TFaceLErr_enum"
  bus_selector_1/37 -> UnitConverter_48/1  "<VINP_TFaceR_C>"
  UnitConverter_48/1 -> bus_creator/48  "VINP_TFaceR_C"
  bus_selector_1/38 -> UnitConverter_49/1  "<VINP_TFaceRErr_enum>"
  UnitConverter_49/1 -> bus_creator/49  "VINP_TFaceRErr_enum"
  bus_selector_1/39 -> UnitConverter_50/1  "<VINP_TFaceRr_C>"
  UnitConverter_50/1 -> bus_creator/50  "VINP_TFaceRr_C"
  bus_selector_1/40 -> UnitConverter_51/1  "<VINP_TFaceRrErr_enum>"
  UnitConverter_51/1 -> bus_creator/51  "VINP_TFaceRrErr_enum"
  bus_selector_1/41 -> UnitConverter_52/1  "<VINP_TFootL_C>"
  UnitConverter_52/1 -> bus_creator/52  "VINP_TFootL_C"
  bus_selector_1/42 -> UnitConverter_53/1  "<VINP_TFootLErr_enum>"
  UnitConverter_53/1 -> bus_creator/53  "VINP_TFootLErr_enum"
  bus_selector_1/43 -> UnitConverter_54/1  "<VINP_TFootR_C>"
  UnitConverter_54/1 -> bus_creator/54  "VINP_TFootR_C"
  bus_selector_1/44 -> UnitConverter_55/1  "<VINP_TFootRErr_enum>"
  UnitConverter_55/1 -> bus_creator/55  "VINP_TFootRErr_enum"
  bus_selector_1/45 -> UnitConverter_56/1  "<VINP_TFootRr_C>"
  UnitConverter_56/1 -> bus_creator/56  "VINP_TFootRr_C"
  bus_selector_1/46 -> UnitConverter_57/1  "<VINP_TFootRrErr_enum>"
  UnitConverter_57/1 -> bus_creator/57  "VINP_TFootRrErr_enum"
  bus_selector_1/47 -> UnitConverter_58/1  "<VINP_Tevap_C>"
  UnitConverter_58/1 -> bus_creator/58  "VINP_Tevap_C"
  bus_selector_1/48 -> UnitConverter_59/1  "<VINP_TevapErr_enum>"
  UnitConverter_59/1 -> bus_creator/59  "VINP_TevapErr_enum"
  bus_selector_1/49 -> UnitConverter_60/1  "<VINP_Tincar_C>"
  UnitConverter_60/1 -> bus_creator/60  "VINP_Tincar_C"
  bus_selector_1/50 -> UnitConverter_61/1  "<VINP_TincarErr_enum>"
  UnitConverter_61/1 -> bus_creator/61  "VINP_TincarErr_enum"
  bus_selector_1/51 -> UnitConverter_62/1  "<VINP_ZoneDrMalfunLevel_enum>"
  UnitConverter_62/1 -> bus_creator/62  "VINP_ZoneDrMalfunLevel_enum"
  bus_selector_1/52 -> UnitConverter_63/1  "<VINP_ChargeInletLockSta_flg>"
  UnitConverter_63/1 -> bus_creator/63  "VINP_ChargeInletLockSta_flg"
  bus_selector_1/53 -> UnitConverter_64/1  "<VINP_CompProEN_flg>"
  UnitConverter_64/1 -> bus_creator/64  "VINP_CompProEN_flg"
  bus_selector_1/54 -> UnitConverter_65/1  "<VINP_FLTurnLampC_mA>"
  UnitConverter_65/1 -> bus_creator/65  "VINP_FLTurnLampC_mA"
  bus_selector_1/55 -> UnitConverter_66/1  "<VINP_FRTurnLampC_mA>"
  UnitConverter_66/1 -> bus_creator/66  "VINP_FRTurnLampC_mA"
  bus_selector_1/56 -> UnitConverter_67/1  "<VINP_FWiperAS_flg>"
  UnitConverter_67/1 -> bus_creator/67  "VINP_FWiperAS_flg"
  bus_selector_1/57 -> UnitConverter_68/1  "<VINP_FWiperProtection_flg>"
  UnitConverter_68/1 -> bus_creator/68  "VINP_FWiperProtection_flg"
  bus_selector_1/58 -> UnitConverter_69/1  "<VINP_TrailerCheck_flg>"
  UnitConverter_69/1 -> bus_creator/69  "VINP_TrailerCheck_flg"
  bus_selector_1/59 -> UnitConverter_70/1  "<VINP_TrailerModeSta_enum>"
  UnitConverter_70/1 -> bus_creator/70  "VINP_TrailerModeSta_enum"
  bus_selector_1/60 -> UnitConverter_71/1  "<VINP_BatInTemp_C>"
  UnitConverter_71/1 -> bus_creator/71  "VINP_BatInTemp_C"
  bus_selector_1/61 -> UnitConverter_72/1  "<VINP_BatInTempErr_enum>"
  UnitConverter_72/1 -> bus_creator/72  "VINP_BatInTempErr_enum"
  bus_selector_1/62 -> UnitConverter_73/1  "<VINP_BatOutTemp_C>"
  UnitConverter_73/1 -> bus_creator/73  "VINP_BatOutTemp_C"
  bus_selector_1/63 -> UnitConverter_74/1  "<VINP_COMPErr_enum>"
  UnitConverter_74/1 -> bus_creator/74  "VINP_COMPErr_enum"
  bus_selector_1/64 -> UnitConverter_75/1  "<VINP_EACProtectEnable_enum>"
  UnitConverter_75/1 -> bus_creator/75  "VINP_EACProtectEnable_enum"
  bus_selector_1/65 -> UnitConverter_76/1  "<VINP_EWP3Err_enum>"
  UnitConverter_76/1 -> bus_creator/76  "VINP_EWP3Err_enum"
  bus_selector_1/66 -> UnitConverter_77/1  "<VINP_EXV1Err_enum>"
  UnitConverter_77/1 -> bus_creator/77  "VINP_EXV1Err_enum"
  bus_selector_1/67 -> UnitConverter_78/1  "<VINP_EXV2Err_enum>"
  UnitConverter_78/1 -> bus_creator/78  "VINP_EXV2Err_enum"
  bus_selector_1/68 -> UnitConverter_79/1  "<VINP_FanErr_enum>"
  UnitConverter_79/1 -> bus_creator/79  "VINP_FanErr_enum"
  bus_selector_1/69 -> UnitConverter_80/1  "<VINP_FrPMMLimpHomeActReq_flg>"
  UnitConverter_80/1 -> bus_creator/80  "VINP_FrPMMLimpHomeActReq_flg"
  bus_selector_1/70 -> UnitConverter_81/1  "<VINP_MotorInTemp_C>"
  UnitConverter_81/1 -> bus_creator/81  "VINP_MotorInTemp_C"
  bus_selector_1/71 -> UnitConverter_82/1  "<VINP_MotorInTempErr_enum>"
  UnitConverter_82/1 -> bus_creator/82  "VINP_MotorInTempErr_enum"
  bus_selector_1/72 -> UnitConverter_83/1  "<VINP_MotorOutTemp_C>"
  UnitConverter_83/1 -> bus_creator/83  "VINP_MotorOutTemp_C"
  bus_selector_1/73 -> UnitConverter_84/1  "<VINP_MotorOutTempErr_enum>"
  UnitConverter_84/1 -> bus_creator/84  "VINP_MotorOutTempErr_enum"
  bus_selector_1/74 -> UnitConverter_85/1  "<VINP_PTHighP_KPa>"
  UnitConverter_85/1 -> bus_creator/85  "VINP_PTHighP_KPa"
  bus_selector_1/75 -> UnitConverter_86/1  "<VINP_PTHighPErr_enum>"
  UnitConverter_86/1 -> bus_creator/86  "VINP_PTHighPErr_enum"
  bus_selector_1/76 -> UnitConverter_87/1  "<VINP_PTHighTact_C>"
  UnitConverter_87/1 -> bus_creator/87  "VINP_PTHighTact_C"
  bus_selector_1/77 -> UnitConverter_88/1  "<VINP_PTHighTactErr_enum>"
  UnitConverter_88/1 -> bus_creator/88  "VINP_PTHighTactErr_enum"
  bus_selector_1/78 -> UnitConverter_89/1  "<VINP_PTLowP1_KPa>"
  UnitConverter_89/1 -> bus_creator/89  "VINP_PTLowP1_KPa"
  bus_selector_1/79 -> UnitConverter_90/1  "<VINP_PTLowP1Err_enum>"
  UnitConverter_90/1 -> bus_creator/90  "VINP_PTLowP1Err_enum"
  bus_selector_1/80 -> UnitConverter_91/1  "<VINP_PTLowP2_KPa>"
  UnitConverter_91/1 -> bus_creator/91  "VINP_PTLowP2_KPa"
  bus_selector_1/81 -> UnitConverter_92/1  "<VINP_PTLowP2Err_enum>"
  UnitConverter_92/1 -> bus_creator/92  "VINP_PTLowP2Err_enum"
  bus_selector_1/82 -> UnitConverter_93/1  "<VINP_PTLowT1_C>"
  UnitConverter_93/1 -> bus_creator/93  "VINP_PTLowT1_C"
  bus_selector_1/83 -> UnitConverter_94/1  "<VINP_PTLowT1Err_enum>"
  UnitConverter_94/1 -> bus_creator/94  "VINP_PTLowT1Err_enum"
  bus_selector_1/84 -> UnitConverter_95/1  "<VINP_PTLowT2_C>"
  UnitConverter_95/1 -> bus_creator/95  "VINP_PTLowT2_C"
  bus_selector_1/85 -> UnitConverter_96/1  "<VINP_PTLowT2Err_enum>"
  UnitConverter_96/1 -> bus_creator/96  "VINP_PTLowT2Err_enum"
  bus_selector_1/86 -> UnitConverter_97/1  "<VINP_SOTXVErr_enum>"
  UnitConverter_97/1 -> bus_creator/97  "VINP_SOTXVErr_enum"
  bus_selector_1/87 -> UnitConverter_98/1  "<VINP_SOV1Err_enum>"
  UnitConverter_98/1 -> bus_creator/98  "VINP_SOV1Err_enum"
  bus_selector_1/88 -> UnitConverter_99/1  "<VINP_SOV2Err_enum>"
  UnitConverter_99/1 -> bus_creator/99  "VINP_SOV2Err_enum"
  bus_selector_1/89 -> UnitConverter_100/1  "<VINP_SOV3Err_enum>"
  UnitConverter_100/1 -> bus_creator/100  "VINP_SOV3Err_enum"
  bus_selector_1/90 -> UnitConverter_101/1  "<VINP_Tamb_C>"
  UnitConverter_101/1 -> bus_creator/101  "VINP_Tamb_C"
  bus_selector_1/91 -> UnitConverter_102/1  "<VINP_TambErr_enum>"
  UnitConverter_102/1 -> bus_creator/102  "VINP_TambErr_enum"
  bus_selector_1/92 -> UnitConverter_103/1  "<VINP_FrntPTCLeActHeatPwr_W>"
  UnitConverter_103/1 -> bus_creator/103  "VINP_FrntPTCLeActHeatPwr_W"
  bus_selector_1/93 -> UnitConverter_104/1  "<VINP_FrntPTCRearLeActHeatPwr_W>"
  UnitConverter_104/1 -> bus_creator/104  "VINP_FrntPTCRearLeActHeatPwr_W"
  bus_selector_1/94 -> UnitConverter_105/1  "<VINP_FrntPTCRearRiActHeatPwr_W>"
  UnitConverter_105/1 -> bus_creator/105  "VINP_FrntPTCRearRiActHeatPwr_W"
  bus_selector_1/95 -> UnitConverter_106/1  "<VINP_FrntPTCRiActHeatPwr_W>"
  UnitConverter_106/1 -> bus_creator/106  "VINP_FrntPTCRiActHeatPwr_W"
  bus_selector_1/96 -> UnitConverter_107/1  "<VINP_COMPActualPwr_W>"
  UnitConverter_107/1 -> bus_creator/107  "VINP_COMPActualPwr_W"
  bus_selector_1/97 -> UnitConverter_108/1  "<VINP_COMPStatorSpd_rpm>"
  UnitConverter_108/1 -> bus_creator/108  "VINP_COMPStatorSpd_rpm"
  bus_selector_1/98 -> UnitConverter_109/1  "<VINP_PTCActuPwrHSC6_enum>"
  UnitConverter_109/1 -> bus_creator/109  "VINP_PTCActuPwrHSC6_enum"
  bus_selector_1/99 -> UnitConverter_110/1  "<VINP_CSWDimSw_flg>"
  UnitConverter_110/1 -> bus_creator/110  "VINP_CSWDimSw_flg"
  bus_selector_1/100 -> UnitConverter_111/1  "<VINP_CSWFWasSwSta_enum>"
  UnitConverter_111/1 -> bus_creator/111  "VINP_CSWFWasSwSta_enum"
  bus_selector_1/101 -> UnitConverter_112/1  "<VINP_CSWFWipSwSta_enum>"
  UnitConverter_112/1 -> bus_creator/112  "VINP_CSWFWipSwSta_enum"
  bus_selector_1/102 -> UnitConverter_113/1  "<VINP_CSWPassSWSta_flg>"
  UnitConverter_113/1 -> bus_creator/113  "VINP_CSWPassSWSta_flg"
  bus_selector_1/103 -> UnitConverter_114/1  "<VINP_CSWRWasSWSta_enum>"
  UnitConverter_114/1 -> bus_creator/114  "VINP_CSWRWasSWSta_enum"
  bus_selector_1/104 -> UnitConverter_115/1  "<VINP_CSWRWipIntSwSta_enum>"
  UnitConverter_115/1 -> bus_creator/115  "VINP_CSWRWipIntSwSta_enum"
  bus_selector_1/105 -> UnitConverter_116/1  "<VINP_CSWTurnSwSta_enum>"
  UnitConverter_116/1 -> bus_creator/116  "VINP_CSWTurnSwSta_enum"
  bus_selector_1/106 -> UnitConverter_117/1  "<VINP_FAPWL01LINResponseError_flg>"
  UnitConverter_117/1 -> bus_creator/117  "VINP_FAPWL01LINResponseError_flg"
  bus_selector_1/107 -> UnitConverter_118/1  "<VINP_LDrvMotorRelayError_flg>"
  UnitConverter_118/1 -> bus_creator/118  "VINP_LDrvMotorRelayError_flg"
  bus_selector_1/108 -> UnitConverter_119/1  "<VINP_LDrvMotorRippleError_flg>"
  UnitConverter_119/1 -> bus_creator/119  "VINP_LDrvMotorRippleError_flg"
  bus_selector_1/109 -> UnitConverter_120/1  "<VINP_LDrvValWdwOpened_pct>"
  UnitConverter_120/1 -> bus_creator/120  "VINP_LDrvValWdwOpened_pct"
  bus_selector_1/110 -> UnitConverter_121/1  "<VINP_LPasMotorRelayError_flg>"
  UnitConverter_121/1 -> bus_creator/121  "VINP_LPasMotorRelayError_flg"
  bus_selector_1/111 -> UnitConverter_122/1  "<VINP_LPasMotorRippleError_flg>"
  UnitConverter_122/1 -> bus_creator/122  "VINP_LPasMotorRippleError_flg"
  bus_selector_1/112 -> UnitConverter_123/1  "<VINP_LPasValWdwOpened_pct>"
  UnitConverter_123/1 -> bus_creator/123  "VINP_LPasValWdwOpened_pct"
  bus_selector_1/113 -> UnitConverter_124/1  "<VINP_LRLDMotorRelayError_flg>"
  UnitConverter_124/1 -> bus_creator/124  "VINP_LRLDMotorRelayError_flg"
  bus_selector_1/114 -> UnitConverter_125/1  "<VINP_LRLDMotorRippleError_flg>"
  UnitConverter_125/1 -> bus_creator/125  "VINP_LRLDMotorRippleError_flg"
  bus_selector_1/115 -> UnitConverter_126/1  "<VINP_LRLDValWdwOpened_pct>"
  UnitConverter_126/1 -> bus_creator/126  "VINP_LRLDValWdwOpened_pct"
  bus_selector_1/116 -> UnitConverter_127/1  "<VINP_LRRDMotorRelayError_flg>"
  UnitConverter_127/1 -> bus_creator/127  "VINP_LRRDMotorRelayError_flg"
  bus_selector_1/117 -> UnitConverter_128/1  "<VINP_LRRDMotorRippleError_flg>"
  UnitConverter_128/1 -> bus_creator/128  "VINP_LRRDMotorRippleError_flg"
  bus_selector_1/118 -> UnitConverter_129/1  "<VINP_LRRDValWdwOpened_pct>"
  UnitConverter_129/1 -> bus_creator/129  "VINP_LRRDValWdwOpened_pct"
  bus_selector_1/119 -> UnitConverter_130/1  "<VINP_RAPWL01LINResponseError_flg>"
  UnitConverter_130/1 -> bus_creator/130  "VINP_RAPWL01LINResponseError_flg"
  bus_selector_1/120 -> UnitConverter_131/1  "<VINP_RLSLampSta_flg>"
  UnitConverter_131/1 -> bus_creator/131  "VINP_RLSLampSta_flg"
  bus_selector_1/121 -> UnitConverter_132/1  "<VINP_RLSRainSnrWiperCmd_enum>"
  UnitConverter_132/1 -> bus_creator/132  "VINP_RLSRainSnrWiperCmd_enum"
  bus_selector_1/122 -> UnitConverter_133/1  "<VINP_SWCACCSta_flg>"
  UnitConverter_133/1 -> bus_creator/133  "VINP_SWCACCSta_flg"
  bus_selector_1/123 -> UnitConverter_134/1  "<VINP_SWCCANCELSta_flg>"
  UnitConverter_134/1 -> bus_creator/134  "VINP_SWCCANCELSta_flg"
  bus_selector_1/124 -> UnitConverter_135/1  "<VINP_SWCDistanceSta_flg>"
  UnitConverter_135/1 -> bus_creator/135  "VINP_SWCDistanceSta_flg"
  bus_selector_1/125 -> UnitConverter_136/1  "<VINP_SWCDownSta_flg>"
  UnitConverter_136/1 -> bus_creator/136  "VINP_SWCDownSta_flg"
  bus_selector_1/126 -> UnitConverter_137/1  "<VINP_SWCLKASta_flg>"
  UnitConverter_137/1 -> bus_creator/137  "VINP_SWCLKASta_flg"
  bus_selector_1/127 -> UnitConverter_138/1  "<VINP_SWCLeftSta_flg>"
  UnitConverter_138/1 -> bus_creator/138  "VINP_SWCLeftSta_flg"
  bus_selector_1/128 -> UnitConverter_139/1  "<VINP_SWCRegenUp_flg>"
  UnitConverter_139/1 -> bus_creator/139  "VINP_SWCRegenUp_flg"
  bus_selector_1/129 -> UnitConverter_140/1  "<VINP_SWCResUpSta_flg>"
  UnitConverter_140/1 -> bus_creator/140  "VINP_SWCResUpSta_flg"
  bus_selector_1/130 -> UnitConverter_141/1  "<VINP_SWCRightSta_flg>"
  UnitConverter_141/1 -> bus_creator/141  "VINP_SWCRightSta_flg"
  bus_selector_1/131 -> UnitConverter_142/1  "<VINP_SWCSetdownSta_flg>"
  UnitConverter_142/1 -> bus_creator/142  "VINP_SWCSetdownSta_flg"
  bus_selector_1/132 -> UnitConverter_143/1  "<VINP_SWCTripSta_flg>"
  UnitConverter_143/1 -> bus_creator/143  "VINP_SWCTripSta_flg"
  bus_selector_1/133 -> UnitConverter_144/1  "<VINP_SWCUndefinedSta_flg>"
  UnitConverter_144/1 -> bus_creator/144  "VINP_SWCUndefinedSta_flg"
  bus_selector_1/134 -> UnitConverter_145/1  "<VINP_SWCUpSta_flg>"
  UnitConverter_145/1 -> bus_creator/145  "VINP_SWCUpSta_flg"
  bus_selector_1/135 -> UnitConverter_146/1  "<VINP_SWCVRSta_flg>"
  UnitConverter_146/1 -> bus_creator/146  "VINP_SWCVRSta_flg"
  bus_selector_1/136 -> UnitConverter_147/1  "<VINP_SWCmodeSta_flg>"
  UnitConverter_147/1 -> bus_creator/147  "VINP_SWCmodeSta_flg"
  [inp_CanValid_bus] -> bus_selector/1
  [inp_Hal_bus] -> bus_selector_1/1
  bus_creator/1 -> BINP_outputs/1
